simulink model "sender"  (R2023a)
settings: Solver=FixedStepAuto  StartTime=0.0  StopTime=10.0  RelTol=1e-3
undefined symbols (not defined in the file): Data_Display, untitled1
libraries: androidcommunicationlib x3, androidaudiovideolib x1, androiduilib x1
settings Model: Creator=ragha  LastModifiedBy=ragha
settings OptimizationCC: EnhancedBackFolding=on  PassReuseOutputArgsAs=Individual arguments  ZeroExternalMemoryAtStartup=off  ZeroInternalMemoryAtStartup=off  MaxStackSize=64  OptimizeBlockOrder=speed  DifferentSizesBufferReuse=on  OptimizationCustomize=off  EfficientTunableParamExpr=on
settings DebuggingCC: ParameterTunabilityLossMsg=error
settings HardwareCC: ProdBitPerPointer=32  ProdBitPerSizeT=32  ProdBitPerPtrDiffT=32  ProdLargestAtomicInteger=Long  ProdLargestAtomicFloat=Double  ProdWordSize=32  ProdHWDeviceType=ARM Compatible->ARM Cortex
settings SFSimCC: MATLABDynamicMemAlloc=off
settings RTWCC: Description=Embedded Coder  SystemTargetFile=ert.tlc  HardwareBoard=Android Device  TLCOptions="-aInlineSetEventsForThisBaseRateFcn=TLC_FALSE -aSuppressMultiTaskScheduler=TLC_FALSE  -aRateBasedStepFcn=0"  TemplateMakefile=ert_default_tmf  RTWVerbose=off  Toolchain=Android SDK/NDK Tools
settings CodeAppCC: ForceParamTrailComments=on  IgnoreCustomStorageClasses=off  OperatorAnnotations=on  SimulinkDataObjDesc=on  SFDataObjDesc=on  InsertBlockDesc=on

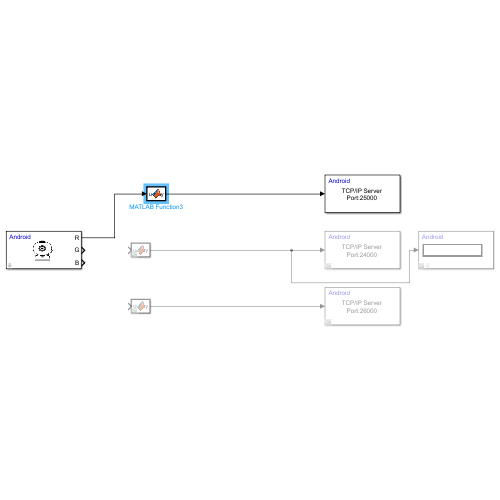
[thumbnail: Simulink's stored preview of the top-level diagram]
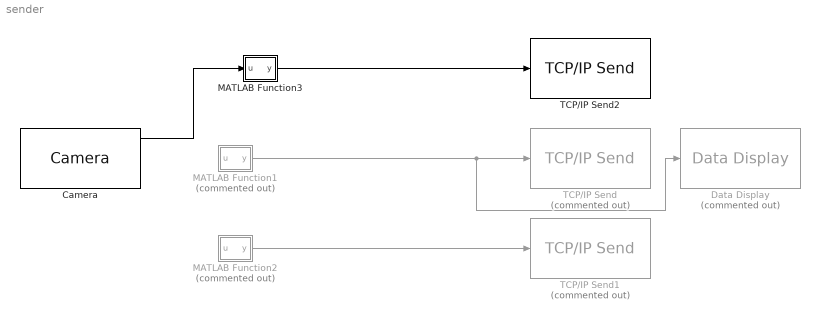
== system sender ==
  Camera : androidaudiovideolib/Camera  CameraLocation=Back  CameraResolutions=Back - 176x144  Width=176  Height=144  SampleTime=0.1  BlockPlatform=Android
  Data Display : androiduilib/Data Display  Commented=on  DataDisplayId=untitled1/Data_Display  Format=Float  Precision=6  SimulateUsing=Code generation  blockPlatform=Android
  MATLAB Function1 : MATLAB Function  Commented=on  TreatAsAtomicUnit=on
  MATLAB Function2 : MATLAB Function  Commented=on  TreatAsAtomicUnit=on
  MATLAB Function3 : MATLAB Function  TreatAsAtomicUnit=on
  TCP/IP Send : androidcommunicationlib/TCP//IP Send  Commented=on  TCPSendId=untitled1/TCP//IP_Send  Mode_=Server  LocalServerPort_=24000  RemoteAddr_=127.0.0.1  RemoteServerPort_=25000  ClientPortBindingSelection_=off  ClientPortToBind_=35000  BlockingMode_=off  BlockTimeout_=1
  TCP/IP Send1 : androidcommunicationlib/TCP//IP Send  Commented=on  TCPSendId=untitled1/TCP//IP_Send1  Mode_=Server  LocalServerPort_=26000  RemoteAddr_=127.0.0.1  RemoteServerPort_=25000  ClientPortBindingSelection_=off  ClientPortToBind_=35000  BlockingMode_=off  BlockTimeout_=1
  TCP/IP Send2 : androidcommunicationlib/TCP//IP Send  TCPSendId=untitled1/TCP//IP_Send2  Mode_=Server  LocalServerPort_=25000  RemoteAddr_=127.0.0.1  RemoteServerPort_=25000  ClientPortBindingSelection_=off  ClientPortToBind_=35000  BlockingMode_=off  BlockTimeout_=1
  wires:
  MATLAB Function1/1(y) -> TCP/IP Send/1, Data Display/1
  MATLAB Function3/1(y) -> TCP/IP Send2/1
  Camera/1 -> MATLAB Function3/1(u)
  MATLAB Function2/1(y) -> TCP/IP Send1/1

== matlab function sender/MATLAB Function3 ==
  data: u input; y output
function y = fcn(u)

y = u;

== matlab function sender/MATLAB Function2 ==
  data: u input; y output
function y = fcn(u)

y = u;

== matlab function sender/MATLAB Function1 ==
  data: u input; y output
function y = fcn(u)

y = u;
